simulink model "Lab3_Topolnitskii_ploop"  (R2021a)
settings: Solver=ode15s  StartTime=0.0  StopTime=1  RelTol=1e-3  EnableMultiTasking=on
undefined symbols (not defined in the file): Amp_noise, Fr_noise, irb140, J, Ki, Kpl, Kv, motor_const, q_end, qz, tau_m
libraries: roblocks x12
settings Model: Creator=pic  LastModifiedBy=Insight
settings SolverCC: AlgebraicLoopSolver=TrustRegion
settings DataIOCC: SaveFormat=Array  SignalLoggingSaveFormat=ModelDataLogs  TimeSaveName=t  OutputSaveName=y  OutputOption=SpecifiedOutputTimes  OutputTimes=[0:0.001:1]'
settings OptimizationCC: ExpressionDepthLimit=2147483647  LifeSpan=inf
settings DebuggingCC: UnderspecifiedInitializationDetection=Classic  MergeDetectMultiDrivingBlocksExec=none  SolverPrmCheckMsg=warning  AllowSymbolicDim=off  StateNameClashWarn=warning  SFUnexpectedBacktrackingDiag=warning  SFNoUnconditionalDefaultTransitionDiag=warning  SFExecutionAtInitializationDiag=none  SFMachineParentedDataDiag=warning  ArithmeticOperatorsInVariantConditions=warning
settings HardwareCC: ProdBitPerPointer=32  ProdBitPerSizeT=32  ProdBitPerPtrDiffT=32  ProdLargestAtomicFloat=None  ProdIntDivRoundTo=Undefined  ProdEndianess=Unspecified  ProdWordSize=32  ProdHWDeviceType=32-bit Generic
settings ModelReferenceCC: PropagateSignalLabelsOutOfModel=off
settings SFSimCC: SimUseLocalCustomCode=off  CustomCodeUndefinedFunction=UseInterfaceOnly
settings RTWCC: RTWUseLocalCustomCode=off
settings CodeAppCC: StateflowObjectComments=on
settings GRTTargetCC: TargetLangStandard=C89/C90 (ANSI)  CombineOutputUpdateFcns=off  GRTInterface=on
settings ConfigComp: CovMetricSettings=dw  CovSaveCumulativeToWorkspaceVar=on  CovSaveSingleToWorkspaceVar=on  CovExternalEMLEnable=off  CovSFcnEnable=off

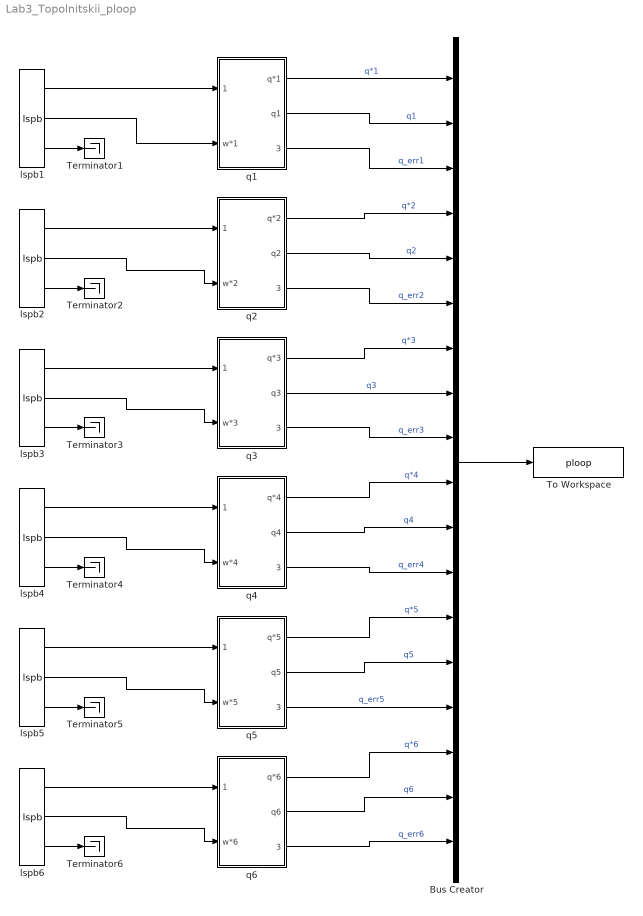
== system Lab3_Topolnitskii_ploop ==
  Bus Creator : BusCreator  Inputs=18
  Terminator{1..6} (6 alike) : Terminator
  To Workspace : ToWorkspace  VariableName=ploop  SaveFormat=Structure With Time  SampleTime=-1
  lspb1 : roblocks/Toolbox/lspb  q0=qz(1)  qf=q_end(1)  tmax=t_end
  lspb2 : roblocks/Toolbox/lspb  q0=qz(2)  qf=q_end(2)  tmax=t_end
  lspb3 : roblocks/Toolbox/lspb  q0=qz(3)  qf=q_end(3)  tmax=t_end
  lspb4 : roblocks/Toolbox/lspb  q0=qz(4)  qf=q_end(4)  tmax=t_end
  lspb5 : roblocks/Toolbox/lspb  q0=qz(5)  qf=q_end(5)  tmax=t_end
  lspb6 : roblocks/Toolbox/lspb  q0=qz(6)  qf=q_end(6)  tmax=t_end
  q1 : Subsystem
  q2 : Subsystem
  q3 : Subsystem
  q4 : Subsystem
  q5 : Subsystem
  q6 : Subsystem
  wires:
  lspb1/1 -> q1/1(theta*1)
  lspb1/3 -> Terminator1/1
  lspb1/2 -> q1/2(w*1)
  lspb2/1 -> q2/1(theta*2)
  lspb2/2 -> q2/2(w*2)
  lspb2/3 -> Terminator2/1
  lspb3/2 -> q3/2(w*3)
  lspb3/3 -> Terminator3/1
  lspb3/1 -> q3/1(theta*3)
  lspb4/2 -> q4/2(w*4)
  lspb4/3 -> Terminator4/1
  lspb4/1 -> q4/1(theta*4)
  lspb5/2 -> q5/2(w*5)
  lspb5/3 -> Terminator5/1
  lspb5/1 -> q5/1(theta*5)
  lspb6/2 -> q6/2(w*6)
  lspb6/3 -> Terminator6/1
  lspb6/1 -> q6/1(theta*6)
  q1/3(q_err1) -> Bus Creator/3  "q_err1"
  q2/3(q_err2) -> Bus Creator/6  "q_err2"
  q3/3(q_err3) -> Bus Creator/9  "q_err3"
  q4/3(q_err4) -> Bus Creator/12  "q_err4"
  q5/3(q_err5) -> Bus Creator/15  "q_err5"
  q6/3(q_err6) -> Bus Creator/18  "q_err6"
  Bus Creator/1 -> To Workspace/1
  q1/1(q*1) -> Bus Creator/1  "q*1"
  q1/2(q1) -> Bus Creator/2  "q1"
  q2/1(q*2) -> Bus Creator/4  "q*2"
  q2/2(q2) -> Bus Creator/5  "q2"
  q3/1(q*3) -> Bus Creator/7  "q*3"
  q3/2(q3) -> Bus Creator/8  "q3"
  q4/1(q*4) -> Bus Creator/10  "q*4"
  q4/2(q4) -> Bus Creator/11  "q4"
  q5/1(q*5) -> Bus Creator/13  "q*5"
  q5/2(q5) -> Bus Creator/14  "q5"
  q6/1(q*6) -> Bus Creator/16  "q*6"
  q6/2(q6) -> Bus Creator/17  "q6"

== system Lab3_Topolnitskii_ploop/q1 ==
  theta*1 : Inport
  w*1 : Inport  Port=2
  Sine Wave : Sin  Amplitude=Amp_noise(1)  Frequency=Fr_noise(1)  SampleTime=0.0001
  Sum : Sum  Inputs=|++
  ploop : Subsystem
  q err : Scope
  "q+q* " : Scope  NumInputPorts=2
  tau_d : Constant  Value=20/107.815
  q*1 : Outport  VectorParamsAs1DForOutWhenUnconnected=off
  q1 : Outport  Port=2  VectorParamsAs1DForOutWhenUnconnected=off
  q_err1 : Outport  Port=3  VectorParamsAs1DForOutWhenUnconnected=off
  wires:
  ploop/2(theta err) -> q_err1/1, q err/1
  tau_d/1 -> Sum/1  "gravity torque"
  theta*1/1 -> "q+q* "/1, q*1/1, ploop/1(theta*)
  ploop/1(theta) -> "q+q* "/2, q1/1  "theta"
  w*1/1 -> ploop/2(w*)
  Sum/1 -> ploop/3(tau_d)
  Sine Wave/1 -> Sum/2

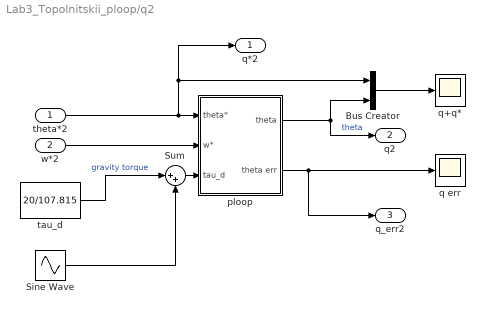
== system Lab3_Topolnitskii_ploop/q2 ==
  theta*2 : Inport
  w*2 : Inport  Port=2
  Bus Creator : BusCreator  Inputs=2
  Sine Wave : Sin  Amplitude=Amp_noise(2)  Frequency=Fr_noise(2)  SampleTime=0.0001
  Sum : Sum  Inputs=|++
  ploop : Subsystem
  q err : Scope
  "q+q* " : Scope
  tau_d : Constant  Value=20/107.815
  q*2 : Outport  VectorParamsAs1DForOutWhenUnconnected=off
  q2 : Outport  Port=2  VectorParamsAs1DForOutWhenUnconnected=off
  q_err2 : Outport  Port=3  VectorParamsAs1DForOutWhenUnconnected=off
  wires:
  ploop/2(theta err) -> q_err2/1, q err/1
  theta*2/1 -> Bus Creator/1, q*2/1, ploop/1(theta*)
  ploop/1(theta) -> q2/1, Bus Creator/2  "theta"
  Bus Creator/1 -> "q+q* "/1
  w*2/1 -> ploop/2(w*)
  Sine Wave/1 -> Sum/2
  tau_d/1 -> Sum/1  "gravity torque"
  Sum/1 -> ploop/3(tau_d)

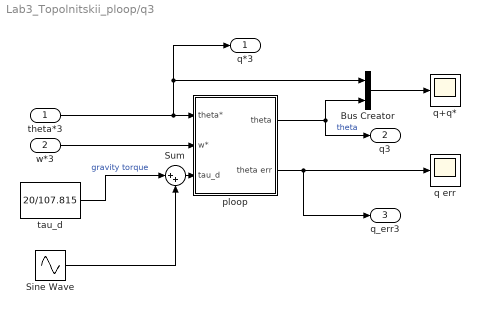
== system Lab3_Topolnitskii_ploop/q3 ==
  theta*3 : Inport
  w*3 : Inport  Port=2
  Bus Creator : BusCreator  Inputs=2
  Sine Wave : Sin  Amplitude=Amp_noise(3)  Frequency=Fr_noise(3)  SampleTime=0.0001
  Sum : Sum  Inputs=|++
  ploop : Subsystem
  q err : Scope
  "q+q* " : Scope
  tau_d : Constant  Value=20/107.815
  q*3 : Outport  VectorParamsAs1DForOutWhenUnconnected=off
  q3 : Outport  Port=2  VectorParamsAs1DForOutWhenUnconnected=off
  q_err3 : Outport  Port=3  VectorParamsAs1DForOutWhenUnconnected=off
  wires:
  ploop/2(theta err) -> q_err3/1, q err/1
  theta*3/1 -> Bus Creator/1, q*3/1, ploop/1(theta*)
  ploop/1(theta) -> q3/1, Bus Creator/2  "theta"
  Bus Creator/1 -> "q+q* "/1
  w*3/1 -> ploop/2(w*)
  Sine Wave/1 -> Sum/2
  tau_d/1 -> Sum/1  "gravity torque"
  Sum/1 -> ploop/3(tau_d)

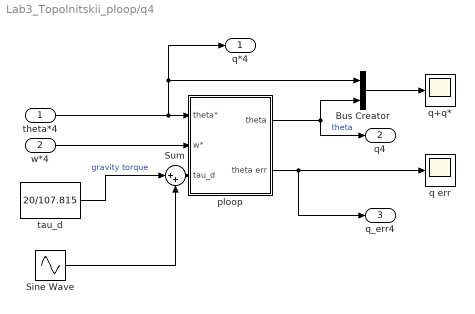
== system Lab3_Topolnitskii_ploop/q4 ==
  theta*4 : Inport
  w*4 : Inport  Port=2
  Bus Creator : BusCreator  Inputs=2
  Sine Wave : Sin  Amplitude=Amp_noise(4)  Frequency=Fr_noise(4)  SampleTime=0.0001
  Sum : Sum  Inputs=|++
  ploop : Subsystem
  q err : Scope
  "q+q* " : Scope
  tau_d : Constant  Value=20/107.815
  q*4 : Outport  VectorParamsAs1DForOutWhenUnconnected=off
  q4 : Outport  Port=2  VectorParamsAs1DForOutWhenUnconnected=off
  q_err4 : Outport  Port=3  VectorParamsAs1DForOutWhenUnconnected=off
  wires:
  ploop/2(theta err) -> q_err4/1, q err/1
  theta*4/1 -> Bus Creator/1, q*4/1, ploop/1(theta*)
  ploop/1(theta) -> q4/1, Bus Creator/2  "theta"
  Bus Creator/1 -> "q+q* "/1
  w*4/1 -> ploop/2(w*)
  Sine Wave/1 -> Sum/2
  tau_d/1 -> Sum/1  "gravity torque"
  Sum/1 -> ploop/3(tau_d)

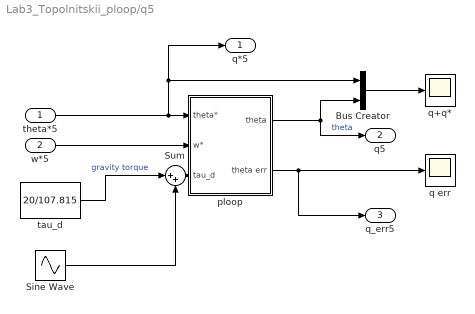
== system Lab3_Topolnitskii_ploop/q5 ==
  theta*5 : Inport
  w*5 : Inport  Port=2
  Bus Creator : BusCreator  Inputs=2
  Sine Wave : Sin  Amplitude=Amp_noise(5)  Frequency=Fr_noise(5)  SampleTime=0.0001
  Sum : Sum  Inputs=|++
  ploop : Subsystem
  q err : Scope
  "q+q* " : Scope
  tau_d : Constant  Value=20/107.815
  q*5 : Outport  VectorParamsAs1DForOutWhenUnconnected=off
  q5 : Outport  Port=2  VectorParamsAs1DForOutWhenUnconnected=off
  q_err5 : Outport  Port=3  VectorParamsAs1DForOutWhenUnconnected=off
  wires:
  ploop/2(theta err) -> q_err5/1, q err/1
  theta*5/1 -> Bus Creator/1, q*5/1, ploop/1(theta*)
  ploop/1(theta) -> q5/1, Bus Creator/2  "theta"
  Bus Creator/1 -> "q+q* "/1
  w*5/1 -> ploop/2(w*)
  Sine Wave/1 -> Sum/2
  tau_d/1 -> Sum/1  "gravity torque"
  Sum/1 -> ploop/3(tau_d)

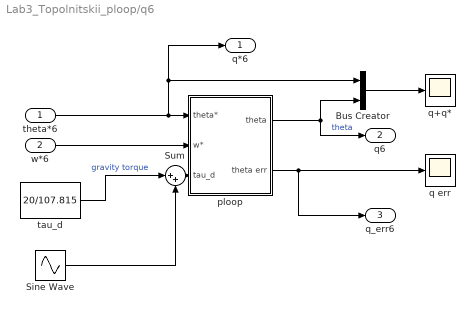
== system Lab3_Topolnitskii_ploop/q6 ==
  theta*6 : Inport
  w*6 : Inport  Port=2
  Bus Creator : BusCreator  Inputs=2
  Sine Wave : Sin  Amplitude=Amp_noise(6)  Frequency=Fr_noise(6)  SampleTime=0.0001
  Sum : Sum  Inputs=|++
  ploop : Subsystem
  q err : Scope
  "q+q* " : Scope
  tau_d : Constant  Value=20/107.815
  q*6 : Outport  VectorParamsAs1DForOutWhenUnconnected=off
  q6 : Outport  Port=2  VectorParamsAs1DForOutWhenUnconnected=off
  q_err6 : Outport  Port=3  VectorParamsAs1DForOutWhenUnconnected=off
  wires:
  ploop/2(theta err) -> q_err6/1, q err/1
  theta*6/1 -> Bus Creator/1, q*6/1, ploop/1(theta*)
  ploop/1(theta) -> q6/1, Bus Creator/2  "theta"
  Bus Creator/1 -> "q+q* "/1
  w*6/1 -> ploop/2(w*)
  Sine Wave/1 -> Sum/2
  tau_d/1 -> Sum/1  "gravity torque"
  Sum/1 -> ploop/3(tau_d)

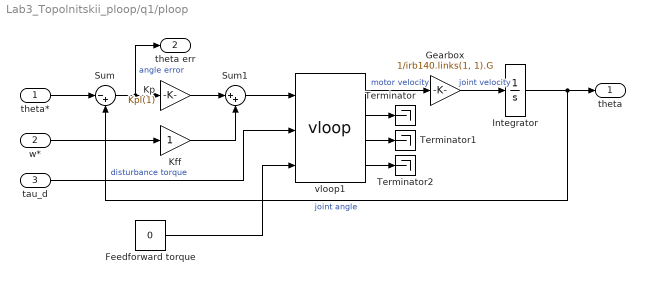
== system Lab3_Topolnitskii_ploop/q1/ploop ==
  theta* : Inport
  w* : Inport  Port=2
  tau_d : Inport  Port=3
  Feedforward torque : Constant  Value=0
  Gearbox : Gain  Gain=1/irb140.links(1, 1).G
  Integrator : Integrator
  Kff : Gain
  Kp : Gain  Gain=Kpl(1)
  Sum : Sum  Inputs=|-+
  Sum1 : Sum  Inputs=|++
  Terminator : Terminator
  Terminator1 : Terminator
  Terminator2 : Terminator
  vloop1 : roblocks/Arm/vloop  J=J(1)  B=irb140.links(1, 1).B  Km=motor_const(1)  tau_max=tau_m(1)  Kv=Kv(1)  Ki=Ki(1)  T=0.0001
  theta : Outport  VectorParamsAs1DForOutWhenUnconnected=off
  theta err : Outport  Port=2  VectorParamsAs1DForOutWhenUnconnected=off
  wires:
  Sum/1 -> Kp/1, theta err/1  "angle error"
  Integrator/1 -> theta/1, Sum/2  "joint angle"
  theta*/1 -> Sum/1
  Kp/1 -> Sum1/1
  Sum1/1 -> vloop1/1
  w*/1 -> Kff/1
  Kff/1 -> Sum1/2
  vloop1/2 -> Terminator/1
  vloop1/3 -> Terminator1/1
  vloop1/4 -> Terminator2/1
  vloop1/1 -> Gearbox/1  "motor velocity"
  tau_d/1 -> vloop1/2  "disturbance torque"
  Feedforward torque/1 -> vloop1/3
  Gearbox/1 -> Integrator/1  "joint velocity"

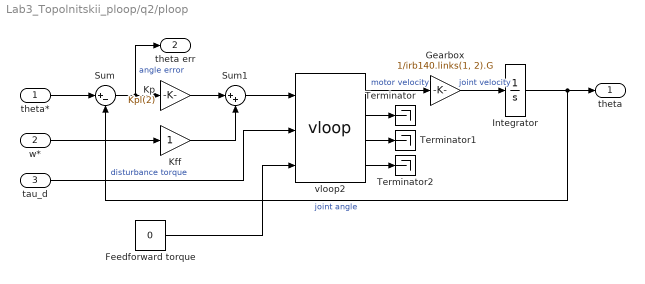
== system Lab3_Topolnitskii_ploop/q2/ploop ==
  theta* : Inport
  w* : Inport  Port=2
  tau_d : Inport  Port=3
  Feedforward torque : Constant  Value=0
  Gearbox : Gain  Gain=1/irb140.links(1, 2).G
  Integrator : Integrator
  Kff : Gain
  Kp : Gain  Gain=Kpl(2)
  Sum : Sum  Inputs=|+-
  Sum1 : Sum  Inputs=|++
  Terminator : Terminator
  Terminator1 : Terminator
  Terminator2 : Terminator
  vloop2 : roblocks/Arm/vloop  J=J(2)  B=irb140.links(1, 2).B  Km=motor_const(2)  tau_max=tau_m(2)  Kv=Kv(2)  Ki=Ki(2)  T=0.0001
  theta : Outport  VectorParamsAs1DForOutWhenUnconnected=off
  theta err : Outport  Port=2  VectorParamsAs1DForOutWhenUnconnected=off
  wires:
  Sum/1 -> Kp/1, theta err/1  "angle error"
  Integrator/1 -> theta/1, Sum/2  "joint angle"
  theta*/1 -> Sum/1
  Kp/1 -> Sum1/1
  Sum1/1 -> vloop2/1
  w*/1 -> Kff/1
  Kff/1 -> Sum1/2
  vloop2/2 -> Terminator/1
  vloop2/3 -> Terminator1/1
  vloop2/4 -> Terminator2/1
  vloop2/1 -> Gearbox/1  "motor velocity"
  tau_d/1 -> vloop2/2  "disturbance torque"
  Feedforward torque/1 -> vloop2/3
  Gearbox/1 -> Integrator/1  "joint velocity"

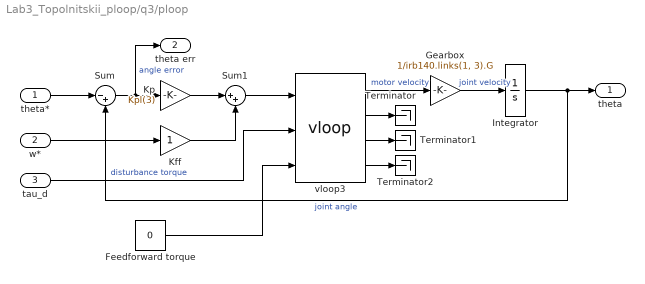
== system Lab3_Topolnitskii_ploop/q3/ploop ==
  theta* : Inport
  w* : Inport  Port=2
  tau_d : Inport  Port=3
  Feedforward torque : Constant  Value=0
  Gearbox : Gain  Gain=1/irb140.links(1, 3).G
  Integrator : Integrator
  Kff : Gain
  Kp : Gain  Gain=Kpl(3)
  Sum : Sum  Inputs=|-+
  Sum1 : Sum  Inputs=|++
  Terminator : Terminator
  Terminator1 : Terminator
  Terminator2 : Terminator
  vloop3 : roblocks/Arm/vloop  J=J(3)  B=irb140.links(1, 3).B  Km=motor_const(3)  tau_max=tau_m(3)  Kv=Kv(3)  Ki=Ki(3)  T=0.0001
  theta : Outport  VectorParamsAs1DForOutWhenUnconnected=off
  theta err : Outport  Port=2  VectorParamsAs1DForOutWhenUnconnected=off
  wires:
  Sum/1 -> Kp/1, theta err/1  "angle error"
  Integrator/1 -> theta/1, Sum/2  "joint angle"
  theta*/1 -> Sum/1
  Kp/1 -> Sum1/1
  Sum1/1 -> vloop3/1
  w*/1 -> Kff/1
  Kff/1 -> Sum1/2
  vloop3/2 -> Terminator/1
  vloop3/3 -> Terminator1/1
  vloop3/4 -> Terminator2/1
  vloop3/1 -> Gearbox/1  "motor velocity"
  tau_d/1 -> vloop3/2  "disturbance torque"
  Feedforward torque/1 -> vloop3/3
  Gearbox/1 -> Integrator/1  "joint velocity"

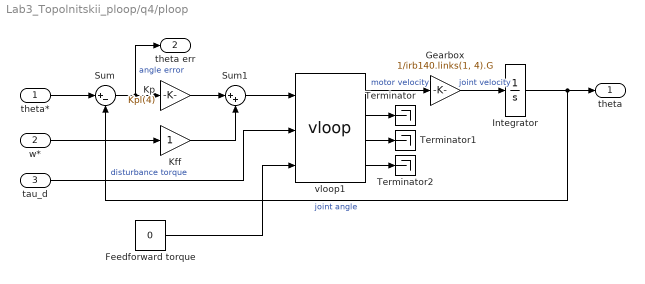
== system Lab3_Topolnitskii_ploop/q4/ploop ==
  theta* : Inport
  w* : Inport  Port=2
  tau_d : Inport  Port=3
  Feedforward torque : Constant  Value=0
  Gearbox : Gain  Gain=1/irb140.links(1, 4).G
  Integrator : Integrator
  Kff : Gain
  Kp : Gain  Gain=Kpl(4)
  Sum : Sum  Inputs=|+-
  Sum1 : Sum  Inputs=|++
  Terminator : Terminator
  Terminator1 : Terminator
  Terminator2 : Terminator
  vloop1 : roblocks/Arm/vloop  J=J(4)  B=irb140.links(1, 4).B  Km=motor_const(4)  tau_max=tau_m(4)  Kv=Kv(4)  Ki=Ki(4)  T=0.0001
  theta : Outport  VectorParamsAs1DForOutWhenUnconnected=off
  theta err : Outport  Port=2  VectorParamsAs1DForOutWhenUnconnected=off
  wires:
  Sum/1 -> Kp/1, theta err/1  "angle error"
  Integrator/1 -> theta/1, Sum/2  "joint angle"
  theta*/1 -> Sum/1
  Kp/1 -> Sum1/1
  Sum1/1 -> vloop1/1
  w*/1 -> Kff/1
  Kff/1 -> Sum1/2
  vloop1/2 -> Terminator/1
  vloop1/3 -> Terminator1/1
  vloop1/4 -> Terminator2/1
  vloop1/1 -> Gearbox/1  "motor velocity"
  tau_d/1 -> vloop1/2  "disturbance torque"
  Feedforward torque/1 -> vloop1/3
  Gearbox/1 -> Integrator/1  "joint velocity"

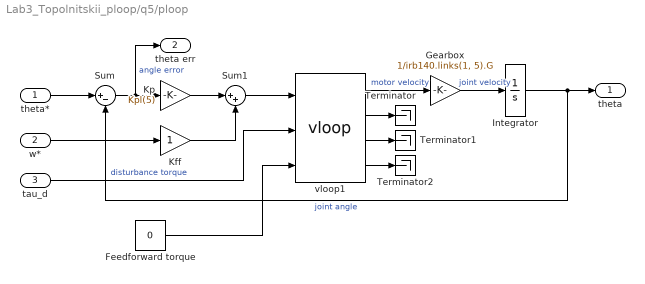
== system Lab3_Topolnitskii_ploop/q5/ploop ==
  theta* : Inport
  w* : Inport  Port=2
  tau_d : Inport  Port=3
  Feedforward torque : Constant  Value=0
  Gearbox : Gain  Gain=1/irb140.links(1, 5).G
  Integrator : Integrator
  Kff : Gain
  Kp : Gain  Gain=Kpl(5)
  Sum : Sum  Inputs=|+-
  Sum1 : Sum  Inputs=|++
  Terminator : Terminator
  Terminator1 : Terminator
  Terminator2 : Terminator
  vloop1 : roblocks/Arm/vloop  J=J(5)  B=irb140.links(1, 5).B  Km=motor_const(5)  tau_max=tau_m(5)  Kv=Kv(5)  Ki=Ki(5)  T=0.0001
  theta : Outport  VectorParamsAs1DForOutWhenUnconnected=off
  theta err : Outport  Port=2  VectorParamsAs1DForOutWhenUnconnected=off
  wires:
  Sum/1 -> Kp/1, theta err/1  "angle error"
  Integrator/1 -> theta/1, Sum/2  "joint angle"
  theta*/1 -> Sum/1
  Kp/1 -> Sum1/1
  Sum1/1 -> vloop1/1
  w*/1 -> Kff/1
  Kff/1 -> Sum1/2
  vloop1/2 -> Terminator/1
  vloop1/3 -> Terminator1/1
  vloop1/4 -> Terminator2/1
  vloop1/1 -> Gearbox/1  "motor velocity"
  tau_d/1 -> vloop1/2  "disturbance torque"
  Feedforward torque/1 -> vloop1/3
  Gearbox/1 -> Integrator/1  "joint velocity"

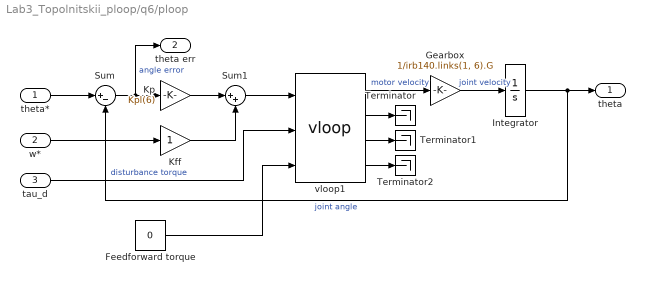
== system Lab3_Topolnitskii_ploop/q6/ploop ==
  theta* : Inport
  w* : Inport  Port=2
  tau_d : Inport  Port=3
  Feedforward torque : Constant  Value=0
  Gearbox : Gain  Gain=1/irb140.links(1, 6).G
  Integrator : Integrator
  Kff : Gain
  Kp : Gain  Gain=Kpl(6)
  Sum : Sum  Inputs=|+-
  Sum1 : Sum  Inputs=|++
  Terminator : Terminator
  Terminator1 : Terminator
  Terminator2 : Terminator
  vloop1 : roblocks/Arm/vloop  J=J(6)  B=irb140.links(1, 6).B  Km=motor_const(6)  tau_max=tau_m(6)  Kv=Kv(6)  Ki=Ki(6)  T=0.0001
  theta : Outport  VectorParamsAs1DForOutWhenUnconnected=off
  theta err : Outport  Port=2  VectorParamsAs1DForOutWhenUnconnected=off
  wires:
  Sum/1 -> Kp/1, theta err/1  "angle error"
  Integrator/1 -> theta/1, Sum/2  "joint angle"
  theta*/1 -> Sum/1
  Kp/1 -> Sum1/1
  Sum1/1 -> vloop1/1
  w*/1 -> Kff/1
  Kff/1 -> Sum1/2
  vloop1/2 -> Terminator/1
  vloop1/3 -> Terminator1/1
  vloop1/4 -> Terminator2/1
  vloop1/1 -> Gearbox/1  "motor velocity"
  tau_d/1 -> vloop1/2  "disturbance torque"
  Feedforward torque/1 -> vloop1/3
  Gearbox/1 -> Integrator/1  "joint velocity"
